simulink model "example1"  (R2014a)
settings: Solver=ode45  StartTime=0.0  StopTime=10.0  RelTol=1e-3
settings Model: Creator=Радион  LastModifiedBy=Радион

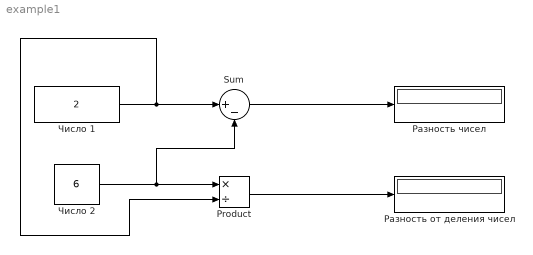
== system example1 ==
  Product : Product  Inputs=*/
  Sum : Sum  Inputs=|+-
  Разность от деления чисел : Display
  Разность чисел : Display
  Число 1 : Constant  Value=2
  Число 2 : Constant  Value=6
  wires:
  Число 2/1 -> Sum/2, Product/1
  Product/1 -> Разность от деления чисел/1
  Sum/1 -> Разность чисел/1
  Число 1/1 -> Product/2, Sum/1
